simulink model "HW1_sim_chaotic_system"  (R2015a)
settings: Solver=ode45  StartTime=0.0  StopTime=60  RelTol=1e-3
settings Model: Creator=123  LastModifiedBy=123

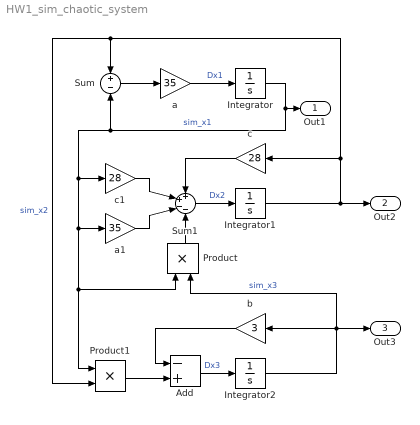
== system HW1_sim_chaotic_system ==
  Add : Sum  Inputs=-+
  Integrator : Integrator  InitialCondition=-10
  Integrator1 : Integrator
  Integrator2 : Integrator  InitialCondition=37
  Product : Product
  Product1 : Product
  Sum : Sum  Inputs=+-
  Sum1 : Sum  Inputs=++--
  a : Gain  Gain=35  OutMax=2
  a1 : Gain  Gain=35  OutMax=2
  b : Gain  Gain=3
  c : Gain  Gain=28
  c1 : Gain  Gain=28
  Out1 : Outport
  Out2 : Outport  Port=2
  Out3 : Outport  Port=3
  wires:
  Integrator1/1 -> Out2/1, c/1, Product1/2, Sum/1  "sim_x2"
  a/1 -> Integrator/1  "Dx1"
  Integrator/1 -> Out1/1, c1/1, Product1/1, Product/1, a1/1, Sum/2  "sim_x1"
  Sum/1 -> a/1
  c/1 -> Sum1/1
  Integrator2/1 -> b/1, Out3/1, Product/2  "sim_x3"
  c1/1 -> Sum1/2
  Product/1 -> Sum1/4
  a1/1 -> Sum1/3
  Sum1/1 -> Integrator1/1  "Dx2"
  b/1 -> Add/1
  Product1/1 -> Add/2
  Add/1 -> Integrator2/1  "Dx3"
